simulink model "GeneralQuadrotorDynamics"  (R2022b)
settings: Solver=VariableStepAuto  StartTime=0.0  StopTime=10.0  RelTol=1e-3
undefined symbols (not defined in the file): rho_0
settings Model: Creator=Baoyi Cui  LastModifiedBy=Baoyi Cui

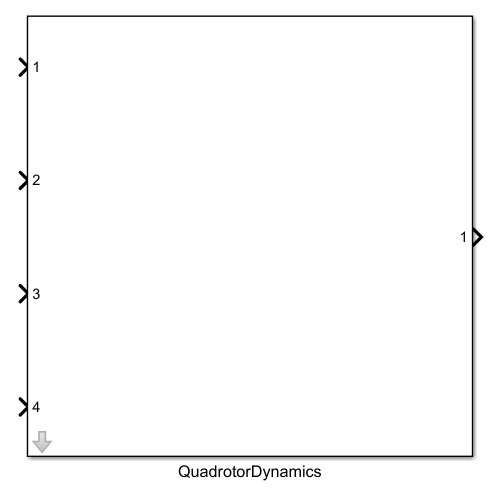
[thumbnail: Simulink's stored preview of the top-level diagram]
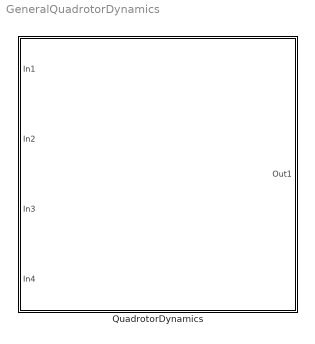
== system GeneralQuadrotorDynamics ==
  QuadrotorDynamics : Subsystem  mask{m=0, g=0, Ixx=0, Iyy=0, Izz=0, L=0, rho=0, gamma=0}
      mask prompts: m "无人机质量"; g "重力加速度"; Ixx "X轴转动惯量"; Iyy "Y轴转动惯量"; Izz "Z轴转动惯量"; L "四旋翼臂长"; rho "四旋翼升力系数"; gamma "空气阻力系数"
      mask DialogControl ParameterGroupVar Prompt: 参数

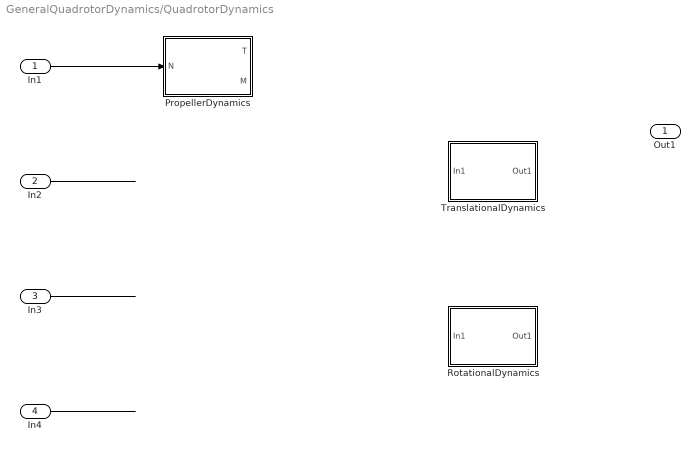
== system GeneralQuadrotorDynamics/QuadrotorDynamics ==
  In1 : Inport
  In2 : Inport  Port=2
  In3 : Inport  Port=3
  In4 : Inport  Port=4
  PropellerDynamics : Subsystem  mask{C_T=0, C_M=0, rho=1.293}
      mask prompts: C_T "拉力系数"; C_M "转矩系数"; rho "飞行环境空气密度(kg/m^3)"
      mask DialogControl ParameterGroupVar Prompt: 参数
  RotationalDynamics : Subsystem
  TranslationalDynamics : Subsystem
  Out1 : Outport
  wires:
  In4/1 -> ?
  In3/1 -> ?
  In2/1 -> ?
  In1/1 -> PropellerDynamics/1(N)

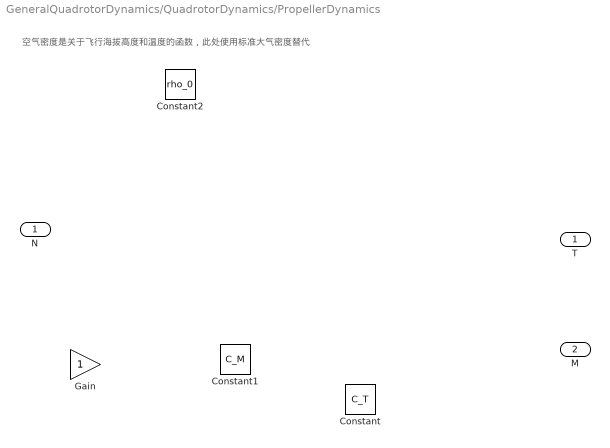
== system GeneralQuadrotorDynamics/QuadrotorDynamics/PropellerDynamics ==
  note: 空气密度是关于飞行海拔高度和温度的函数，此处使用标准大气密度替代
  N : Inport
  Constant : Constant  Value=C_T
  Constant1 : Constant  Value=C_M
  Constant2 : Constant  Value=rho_0
  Gain : Gain
  T : Outport
  M : Outport  Port=2

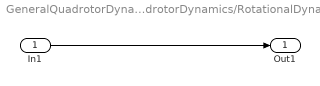
== system GeneralQuadrotorDynamics/QuadrotorDynamics/RotationalDynamics ==
  In1 : Inport
  Out1 : Outport
  wires:
  In1/1 -> Out1/1

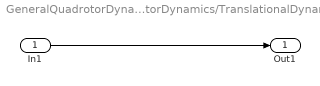
== system GeneralQuadrotorDynamics/QuadrotorDynamics/TranslationalDynamics ==
  In1 : Inport
  Out1 : Outport
  wires:
  In1/1 -> Out1/1
